simulink model "Aufgabe_5_2_3_Timer"  (R2023b)
settings: Solver=ode3  StartTime=0.0  StopTime=10.0  FixedStep=0.01  RelTol=1e-3  EnableMultiTasking=on
settings Model: Creator=JCP  LastModifiedBy=JCP

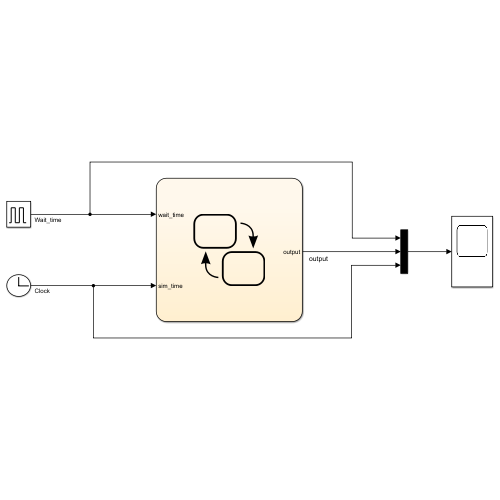
[thumbnail: Simulink's stored preview of the top-level diagram]
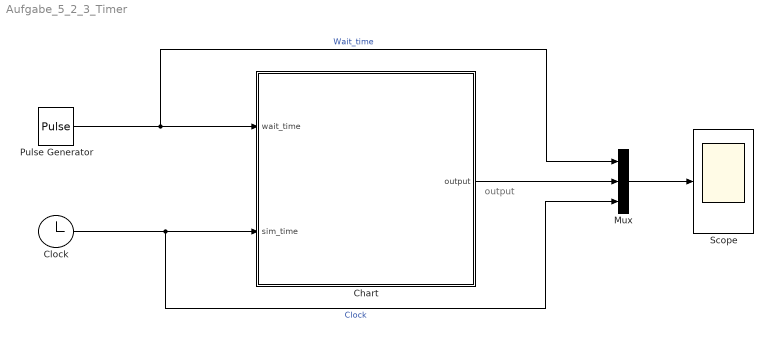
== system Aufgabe_5_2_3_Timer ==
  note: output
  Chart : Stateflow chart  TreatAsAtomicUnit=on
  Clock : Clock
  Mux : Mux  Inputs=3
  Pulse Generator : DiscretePulseGenerator  PulseType=Time based  Period=3  PulseWidth=50
  Scope : Scope
  wires:
  Pulse Generator/1 -> Mux/1, Chart/1(wait_time)  "Wait_time"
  Clock/1 -> Mux/3, Chart/2(sim_time)  "Clock"
  Chart/1(output) -> Mux/2
  Mux/1 -> Scope/1

== stateflow chart Aufgabe_5_2_3_Timer/Chart ==
  state Timer
    state start
      entry: output = 0;
    state wait
      entry: warten = wait_time;
      entry: start_time = sim_time;
    state check
      entry: output = 1;
    (default) -> start
    start -> wait : [wait_time ~= 0]
    check -> start
    wait -> check : [(sim_time - start_time) >=  (warten)]
  data: output output; wait_time input; sim_time input; start_time local; warten local
